simulink model "HalfBridgeRD"  (R2016a)
settings: Solver=VariableStepAuto  StartTime=0.0  StopTime=1.4e-6  RelTol=1e-3
values from neighbouring files (symbols this model uses):
  Dbot = 49    [HalfBridgeRDS.m]
  DelayBot = 50    [HalfBridgeRDS.m]
  DelayTop = 0    [HalfBridgeRDS.m]
  Dtop = 49    [HalfBridgeRDS.m]
  fsw = 1000e3    (= 1000000)    [HalfBridgeRDS.m]
  Rd = 25e-6    (= 2.5e-05)    [HalfBridgeRDS.m]
  Rg = 1    [HalfBridgeRDS.m]
  Rload = 10    [HalfBridgeRDS.m]
  Roff = 2    [HalfBridgeRDS.m]
  Ron = 12    [HalfBridgeRDS.m]
  Rs = 25e-6    (= 2.5e-05)    [HalfBridgeRDS.m]
libraries: elec_lib x28, fl_lib x14, nesl_utility x14
settings Model: Creator=ugurm  LastModifiedBy=ugurm

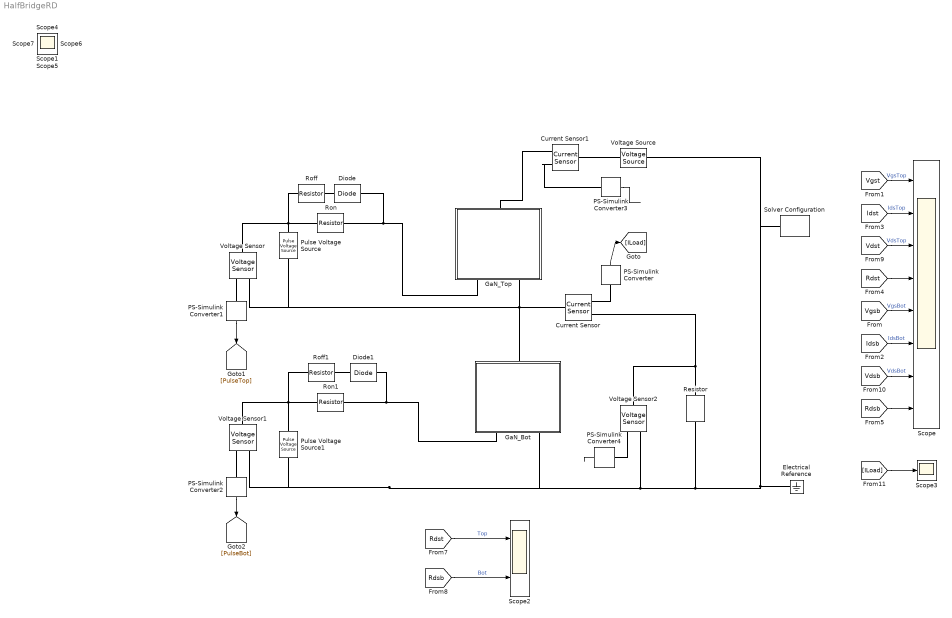
== system HalfBridgeRD ==
  Current Sensor : fl_lib/Electrical/Electrical Sensors/Current Sensor
  Current Sensor1 : fl_lib/Electrical/Electrical Sensors/Current Sensor
  Diode : elec_lib/Semiconductor Devices/Diode  ModelType=1  Vf=0.6 V  Ron=0.3 Ohm  Goff=1e-8 S  Rz=0.3 Ohm  Vz=50 V  C_PWL=5 pF  prmExp=1  I12=[ 0.0137 0.545 ] A  V12=[ 0.6 0.7 ] V  I1=0.0137 A  V1=0.6 V  RS=0.01 Ohm  IS=1e-12 A  Tmeas=25 degC  ec=1  BV=Inf V  C_param=1  CJ0=5 pF  VJ=1 V  Mgrad=0.5  Vvec=[ 0.1 10 100 ] V  Cvec=[ 3.5 1 0.4 ] pF  FC=0.5  Q_param=1  Irrm=-7.15 A  iF=4 A  didt=-750 A/us  trr=115 ns  TT=50 ns  tau=100 ns  T_param=1  IS_T2=1.25e-7 A  I1_T2=0.245 A  V1_T2=0.5 V  Tmeas2=125 degC  EG_param=1  EG=1.11 eV  XTI_param=1  XTI=3  dBVdT=0 V/K  Tdevice=25 degC  Rth=[ 0 10 ] K/W  thermal_mass_parameterization=1  thermal_mass=[ 0 1 ] J/K  thermal_time_constant=[ 0 10 ] s  thermal_mass_initial_temperatures=[ 25 25 ] degC
  Diode1 : elec_lib/Semiconductor Devices/Diode  ModelType=1  Vf=0.6 V  Ron=0.3 Ohm  Goff=1e-8 S  Rz=0.3 Ohm  Vz=50 V  C_PWL=5 pF  prmExp=1  I12=[ 0.0137 0.545 ] A  V12=[ 0.6 0.7 ] V  I1=0.0137 A  V1=0.6 V  RS=0.01 Ohm  IS=1e-12 A  Tmeas=25 degC  ec=1  BV=Inf V  C_param=1  CJ0=5 pF  VJ=1 V  Mgrad=0.5  Vvec=[ 0.1 10 100 ] V  Cvec=[ 3.5 1 0.4 ] pF  FC=0.5  Q_param=1  Irrm=-7.15 A  iF=4 A  didt=-750 A/us  trr=115 ns  TT=50 ns  tau=100 ns  T_param=1  IS_T2=1.25e-7 A  I1_T2=0.245 A  V1_T2=0.5 V  Tmeas2=125 degC  EG_param=1  EG=1.11 eV  XTI_param=1  XTI=3  dBVdT=0 V/K  Tdevice=25 degC  Rth=[ 0 10 ] K/W  thermal_mass_parameterization=1  thermal_mass=[ 0 1 ] J/K  thermal_time_constant=[ 0 10 ] s  thermal_mass_initial_temperatures=[ 25 25 ] degC
  Electrical Reference : fl_lib/Electrical/Electrical Elements/Electrical Reference
  GaN_Bot : Subsystem
  GaN_Top : Subsystem
  PS-Simulink Converter{,1..4} (5 alike) : nesl_utility/PS-Simulink Converter  PhysicalDomain=network_engine_domain  SubClassName=ps_output  LeftPortType=input  RightPortType=output  PseudoPeriodic=off  Frequencies=[]  Unit=1  AffineConversion=off
  Pulse Voltage Source : elec_lib/Additional Components/SPICE-Compatible Components/Sources/Pulse Voltage Source  V1=-3 V  V2=PulseAmplitude V  TD=DelayTop/(100*fsw) s  TR=1e-9 s  TF=1e-9 s  PW=Dtop/(100*fsw) s  PER=1/fsw s
  Pulse Voltage Source1 : elec_lib/Additional Components/SPICE-Compatible Components/Sources/Pulse Voltage Source  V1=-3 V  V2=PulseAmplitude V  TD=DelayBot/(100*fsw) s  TR=1e-9 s  TF=1e-9 s  PW=Dbot/(100*fsw) s  PER=1/fsw s
  Resistor : elec_lib/Passive Devices/Resistor  R=Rload Ohm  R_tol=5  enable_R_tol=0  tol_distribution=1  nSigma=4  enable_operating_limits=0  operating_limit_action=2  max_working_voltage=100 V  power_rating=1 W  enable_faults=0  fault_action=1  R_faulted=Inf Ohm  enable_temporal_fault=0  t_fault=1 s  enable_behavioral_fault=0  max_permissible_current=1 A  t_fail_on_current=1 s  noise_mode=0  sample_time=0.001 s  repeatability=1  auto_seed=3802589887  user_seed=0  Tdevice=25 degC  alpha=0.00393 1/K  Tmeas=25 degC  thermal_mass=100 J/K  initial_temperature=25 degC  power_derating_T1=70 degC  power_derating_T2=155 degC  operating_temperature_range_vec=[ -50 150 ] degC
  Roff : elec_lib/Passive Devices/Resistor  R=Roff Ohm  R_tol=5  enable_R_tol=0  tol_distribution=1  nSigma=4  enable_operating_limits=0  operating_limit_action=2  max_working_voltage=100 V  power_rating=1 W  enable_faults=0  fault_action=1  R_faulted=Inf Ohm  enable_temporal_fault=0  t_fault=1 s  enable_behavioral_fault=0  max_permissible_current=1 A  t_fail_on_current=1 s  noise_mode=0  sample_time=0.001 s  repeatability=1  auto_seed=935450722  user_seed=0  Tdevice=25 degC  alpha=0.00393 1/K  Tmeas=25 degC  thermal_mass=100 J/K  initial_temperature=25 degC  power_derating_T1=70 degC  power_derating_T2=155 degC  operating_temperature_range_vec=[ -50 150 ] degC
  Roff1 : elec_lib/Passive Devices/Resistor  R=Roff Ohm  R_tol=5  enable_R_tol=0  tol_distribution=1  nSigma=4  enable_operating_limits=0  operating_limit_action=2  max_working_voltage=100 V  power_rating=1 W  enable_faults=0  fault_action=1  R_faulted=Inf Ohm  enable_temporal_fault=0  t_fault=1 s  enable_behavioral_fault=0  max_permissible_current=1 A  t_fail_on_current=1 s  noise_mode=0  sample_time=0.001 s  repeatability=1  auto_seed=1550577895  user_seed=0  Tdevice=25 degC  alpha=0.00393 1/K  Tmeas=25 degC  thermal_mass=100 J/K  initial_temperature=25 degC  power_derating_T1=70 degC  power_derating_T2=155 degC  operating_temperature_range_vec=[ -50 150 ] degC
  Ron : elec_lib/Passive Devices/Resistor  R=Ron Ohm  R_tol=5  enable_R_tol=0  tol_distribution=1  nSigma=4  enable_operating_limits=0  operating_limit_action=2  max_working_voltage=100 V  power_rating=1 W  enable_faults=0  fault_action=1  R_faulted=Inf Ohm  enable_temporal_fault=0  t_fault=1 s  enable_behavioral_fault=0  max_permissible_current=1 A  t_fail_on_current=1 s  noise_mode=0  sample_time=0.001 s  repeatability=1  auto_seed=782289965  user_seed=0  Tdevice=25 degC  alpha=0.00393 1/K  Tmeas=25 degC  thermal_mass=100 J/K  initial_temperature=25 degC  power_derating_T1=70 degC  power_derating_T2=155 degC  operating_temperature_range_vec=[ -50 150 ] degC
  Ron1 : elec_lib/Passive Devices/Resistor  R=Ron Ohm  R_tol=5  enable_R_tol=0  tol_distribution=1  nSigma=4  enable_operating_limits=0  operating_limit_action=2  max_working_voltage=100 V  power_rating=1 W  enable_faults=0  fault_action=1  R_faulted=Inf Ohm  enable_temporal_fault=0  t_fault=1 s  enable_behavioral_fault=0  max_permissible_current=1 A  t_fail_on_current=1 s  noise_mode=0  sample_time=0.001 s  repeatability=1  auto_seed=2664075559  user_seed=0  Tdevice=25 degC  alpha=0.00393 1/K  Tmeas=25 degC  thermal_mass=100 J/K  initial_temperature=25 degC  power_derating_T1=70 degC  power_derating_T2=155 degC  operating_temperature_range_vec=[ -50 150 ] degC
  Scope : Scope  NumInputPorts=8
  Scope2 : Scope  NumInputPorts=2
  Scope{1,3..7} (6 alike) : Scope
  Solver Configuration : nesl_utility/Solver Configuration  PhysicalDomain=network_engine_domain  SubClassName=solver  LeftPortType=input  RightPortType=generic  Accelerate=off  Tones=[]  Harmonics=[]  SimulateNoise=off  Profile=off  UseLocalSampling=off  EnableSwitchedLinearOptims=on  FrequencyDomain=off  UseCCode=off  RelTol=0.001  AbsTol=1e-06  MinStep=1e-09  ToWorkspace=off  RevertToSquareIcSolve=off  NumHomotopyIterations=100  PhasorMode=off  PhasorModeNumHarmonics=1  OverrideAbsTol=off  DoDC=off  ResidualTolerance=1e-09  UseLocalSolver=on  LocalSolverChoice=NE_BACKWARD_EULER_ADVANCER  LocalSolverSampleTime=SampleTime  DoFixedCost=on  MaxNonlinIter=3  MaxModeIter=2  LinearAlgebra=Sparse  DelaysMemoryBudget=1024  AutomaticFiltering=on  FilteringTimeConstant=0.001
  Voltage Sensor : fl_lib/Electrical/Electrical Sensors/Voltage Sensor
  Voltage Sensor1 : fl_lib/Electrical/Electrical Sensors/Voltage Sensor
  Voltage Sensor2 : fl_lib/Electrical/Electrical Sensors/Voltage Sensor
  Voltage Source : elec_lib/Sources/Voltage Source  dc_voltage=Vdc V  ac_voltage=0 V  ac_shift=0 deg  ac_frequency=60 Hz  noise_mode=0  PSD=0 V^2/Hz  sample_time=0.001 s  repeatability=1  auto_seed=79941259  user_seed=0
  wires:
  PS-Simulink Converter/1 -> [ILoad]
  PS-Simulink Converter1/1 -> [PulseTop]
  PS-Simulink Converter2/1 -> [PulseBot]
  [Rdst] -> Scope2/1  "Top"
  [Rdsb] -> Scope2/2  "Bot"
  [Idst] -> Scope/2  "IdsTop"
  [Vgst] -> Scope/1  "VgsTop"
  [Vdst] -> Scope/3  "VdsTop"
  [ILoad] -> Scope3/1
  PS-Simulink Converter3/1 -> ?
  PS-Simulink Converter4/1 -> ?
  [Vgsb] -> Scope/5  "VgsBot"
  [Idsb] -> Scope/6  "IdsBot"
  [Vdsb] -> Scope/7  "VdsBot"
  [Rdst] -> Scope/4
  [Rdsb] -> Scope/8
  connections:
  Roff/RConn1 -- Ron/RConn1 -- Voltage Sensor/LConn1 -- Pulse Voltage Source/LConn1
  Diode/LConn1 -- Ron/LConn1 -- GaN_Top/LConn1
  Roff/LConn1 -- Diode/RConn1
  GaN_Top/LConn2 -- GaN_Bot/RConn1 -- Current Sensor/LConn1 -- Voltage Sensor/RConn2 -- Pulse Voltage Source/RConn1
  Pulse Voltage Source1/LConn1 -- Voltage Sensor1/LConn1 -- Ron1/RConn1 -- Roff1/RConn1
  Diode1/LConn1 -- GaN_Bot/LConn1 -- Ron1/LConn1
  Roff1/LConn1 -- Diode1/RConn1
  GaN_Bot/LConn2 -- Voltage Sensor1/RConn2 -- Pulse Voltage Source1/RConn1 -- Electrical Reference/LConn1 -- Voltage Source/RConn1 -- Solver Configuration/RConn1 -- Resistor/RConn1 -- Voltage Sensor2/RConn2
  PS-Simulink Converter/LConn1 -- Current Sensor/RConn1
  PS-Simulink Converter1/LConn1 -- Voltage Sensor/RConn1
  PS-Simulink Converter2/LConn1 -- Voltage Sensor1/RConn1
  Resistor/LConn1 -- Voltage Sensor2/LConn1 -- Current Sensor/RConn2
  Current Sensor1/RConn1 -- PS-Simulink Converter3/LConn1
  Voltage Sensor2/RConn1 -- PS-Simulink Converter4/LConn1
  Current Sensor1/RConn2 -- GaN_Top/RConn1
  Current Sensor1/LConn1 -- Voltage Source/LConn1

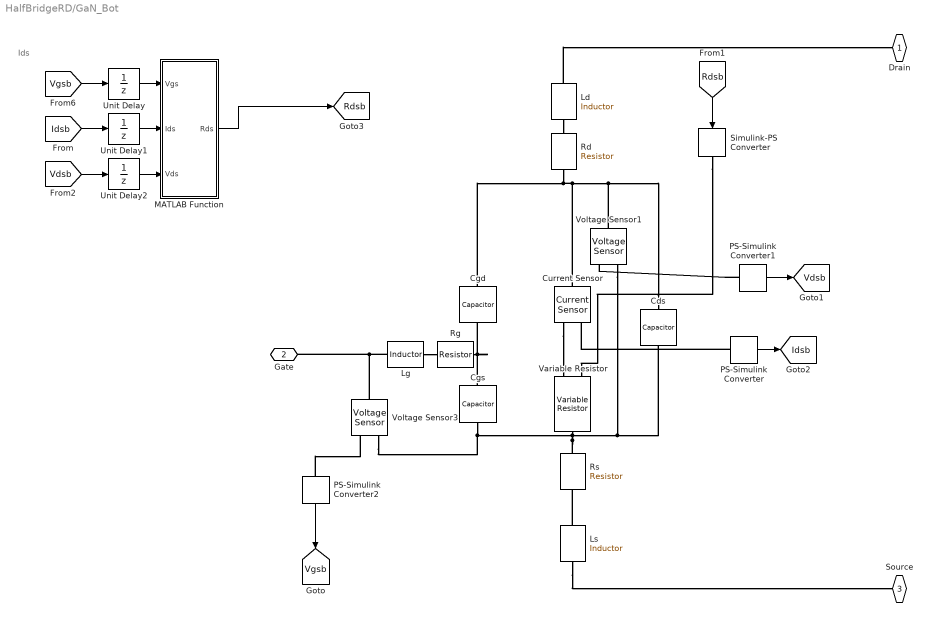
== system HalfBridgeRD/GaN_Bot ==
  note: Ids
  Cds : elec_lib/Passive Devices/Capacitor  enable_table=0  c=Cds F  Cvec=[ 1e-5 1e-6 ] F  Vvec=[ 0 10 ] V  CV_table_symmetry=1  C_tol=5  enable_C_tol=0  tol_distribution=1  nSigma=4  r=1e-6 Ohm  g=0 1/Ohm  initV=0 V  enable_operating_limits=0  operating_limit_action=2  max_working_voltage_range=[ -25 25 ] V  power_rating=1 W  enable_faults=0  fault_action=1  Cscale_faulted=100  R_faulted=0.001 Ohm  G_faulted=0 1/Ohm  tau_fault=0.001 s  enable_temporal_fault=0  t_fault=1 s  enable_behavioral_fault=0  max_permissible_voltage_range=[ -100 100 ] V  t_fail_on_voltage=1 s
  Cgd : elec_lib/Passive Devices/Capacitor  enable_table=0  c=Cgd F  Cvec=[ 1e-5 1e-6 ] F  Vvec=[ 0 10 ] V  CV_table_symmetry=1  C_tol=5  enable_C_tol=0  tol_distribution=1  nSigma=4  r=1e-6 Ohm  g=0 1/Ohm  initV=0 V  enable_operating_limits=0  operating_limit_action=2  max_working_voltage_range=[ -25 25 ] V  power_rating=1 W  enable_faults=0  fault_action=1  Cscale_faulted=100  R_faulted=0.001 Ohm  G_faulted=0 1/Ohm  tau_fault=0.001 s  enable_temporal_fault=0  t_fault=1 s  enable_behavioral_fault=0  max_permissible_voltage_range=[ -100 100 ] V  t_fail_on_voltage=1 s
  Cgs : elec_lib/Passive Devices/Capacitor  enable_table=0  c=Cgs F  Cvec=[ 1e-5 1e-6 ] F  Vvec=[ 0 10 ] V  CV_table_symmetry=1  C_tol=5  enable_C_tol=0  tol_distribution=1  nSigma=4  r=1e-6 Ohm  g=0 1/Ohm  initV=0 V  enable_operating_limits=0  operating_limit_action=2  max_working_voltage_range=[ -25 25 ] V  power_rating=1 W  enable_faults=0  fault_action=1  Cscale_faulted=100  R_faulted=0.001 Ohm  G_faulted=0 1/Ohm  tau_fault=0.001 s  enable_temporal_fault=0  t_fault=1 s  enable_behavioral_fault=0  max_permissible_voltage_range=[ -100 100 ] V  t_fail_on_voltage=1 s
  Current Sensor : fl_lib/Electrical/Electrical Sensors/Current Sensor
  Ld : elec_lib/Passive Devices/Inductor  l=Ld H  L_tol=5  enable_L_tol=0  tol_distribution=1  nSigma=4  r=0 Ohm  g=1e-9 1/Ohm  initI=0 A  enable_operating_limits=0  operating_limit_action=2  max_working_current=1 A  power_rating=1 W  enable_faults=0  fault_action=1  lambdaPercent=50  k_faulted=0.9999 Ohm  turnsShort=0  openCct=0  groundShort=0  groundShortG=0 1/Ohm  tau_fault=0.001 s  enable_temporal_fault=0  t_fault=1 s  enable_behavioral_fault=0  max_permissible_voltage=100 V  n_fail_on_voltage=1  max_permissible_current=1 A  t_fail_on_current=1 s
  Lg : elec_lib/Passive Devices/Inductor  l=Lg H  L_tol=5  enable_L_tol=0  tol_distribution=1  nSigma=4  r=0 Ohm  g=1e-9 1/Ohm  initI=0 A  enable_operating_limits=0  operating_limit_action=2  max_working_current=1 A  power_rating=1 W  enable_faults=0  fault_action=1  lambdaPercent=50  k_faulted=0.9999 Ohm  turnsShort=0  openCct=0  groundShort=0  groundShortG=0 1/Ohm  tau_fault=0.001 s  enable_temporal_fault=0  t_fault=1 s  enable_behavioral_fault=0  max_permissible_voltage=100 V  n_fail_on_voltage=1  max_permissible_current=1 A  t_fail_on_current=1 s
  Ls : elec_lib/Passive Devices/Inductor  l=Ls H  L_tol=5  enable_L_tol=0  tol_distribution=1  nSigma=4  r=0 Ohm  g=1e-9 1/Ohm  initI=0 A  enable_operating_limits=0  operating_limit_action=2  max_working_current=1 A  power_rating=1 W  enable_faults=0  fault_action=1  lambdaPercent=50  k_faulted=0.9999 Ohm  turnsShort=0  openCct=0  groundShort=0  groundShortG=0 1/Ohm  tau_fault=0.001 s  enable_temporal_fault=0  t_fault=1 s  enable_behavioral_fault=0  max_permissible_voltage=100 V  n_fail_on_voltage=1  max_permissible_current=1 A  t_fail_on_current=1 s
  MATLAB Function : MATLAB Function  TreatAsAtomicUnit=on
  PS-Simulink Converter : nesl_utility/PS-Simulink Converter  PhysicalDomain=network_engine_domain  SubClassName=ps_output  LeftPortType=input  RightPortType=output  PseudoPeriodic=off  Frequencies=[]  Unit=1  AffineConversion=off
  PS-Simulink Converter1 : nesl_utility/PS-Simulink Converter  PhysicalDomain=network_engine_domain  SubClassName=ps_output  LeftPortType=input  RightPortType=output  PseudoPeriodic=off  Frequencies=[]  Unit=1  AffineConversion=off
  PS-Simulink Converter2 : nesl_utility/PS-Simulink Converter  PhysicalDomain=network_engine_domain  SubClassName=ps_output  LeftPortType=input  RightPortType=output  PseudoPeriodic=off  Frequencies=[]  Unit=1  AffineConversion=off
  Rd : elec_lib/Passive Devices/Resistor  R=Rd Ohm  R_tol=5  enable_R_tol=0  tol_distribution=1  nSigma=4  enable_operating_limits=0  operating_limit_action=2  max_working_voltage=100 V  power_rating=1 W  enable_faults=0  fault_action=1  R_faulted=Inf Ohm  enable_temporal_fault=0  t_fault=1 s  enable_behavioral_fault=0  max_permissible_current=1 A  t_fail_on_current=1 s  noise_mode=0  sample_time=0.001 s  repeatability=1  auto_seed=2598415021  user_seed=0  Tdevice=25 degC  alpha=0.00393 1/K  Tmeas=25 degC  thermal_mass=100 J/K  initial_temperature=25 degC  power_derating_T1=70 degC  power_derating_T2=155 degC  operating_temperature_range_vec=[ -50 150 ] degC
  Rg : elec_lib/Passive Devices/Resistor  R=Rg Ohm  R_tol=5  enable_R_tol=0  tol_distribution=1  nSigma=4  enable_operating_limits=0  operating_limit_action=2  max_working_voltage=100 V  power_rating=1 W  enable_faults=0  fault_action=1  R_faulted=Inf Ohm  enable_temporal_fault=0  t_fault=1 s  enable_behavioral_fault=0  max_permissible_current=1 A  t_fail_on_current=1 s  noise_mode=0  sample_time=0.001 s  repeatability=1  auto_seed=1663206464  user_seed=0  Tdevice=25 degC  alpha=0.00393 1/K  Tmeas=25 degC  thermal_mass=100 J/K  initial_temperature=25 degC  power_derating_T1=70 degC  power_derating_T2=155 degC  operating_temperature_range_vec=[ -50 150 ] degC
  Rs : elec_lib/Passive Devices/Resistor  R=Rs Ohm  R_tol=5  enable_R_tol=0  tol_distribution=1  nSigma=4  enable_operating_limits=0  operating_limit_action=2  max_working_voltage=100 V  power_rating=1 W  enable_faults=0  fault_action=1  R_faulted=Inf Ohm  enable_temporal_fault=0  t_fault=1 s  enable_behavioral_fault=0  max_permissible_current=1 A  t_fail_on_current=1 s  noise_mode=0  sample_time=0.001 s  repeatability=1  auto_seed=610689199  user_seed=0  Tdevice=25 degC  alpha=0.00393 1/K  Tmeas=25 degC  thermal_mass=100 J/K  initial_temperature=25 degC  power_derating_T1=70 degC  power_derating_T2=155 degC  operating_temperature_range_vec=[ -50 150 ] degC
  Simulink-PS Converter : nesl_utility/Simulink-PS Converter  PhysicalDomain=network_engine_domain  SubClassName=ps_input  LeftPortType=input  RightPortType=output  PseudoPeriodic=off  Frequencies=[]  NoiseDistribution=none  NoiseParameters=[]  Unit=1  AffineConversion=off  InputFiltering=off  SimscapeFilterOrder=1  InputFilterTimeConstant=0.001  UdotUserProvided=1
  Unit Delay : UnitDelay  SampleTime=-1
  Unit Delay1 : UnitDelay  SampleTime=-1
  Unit Delay2 : UnitDelay  InitialCondition=1  SampleTime=-1
  Variable Resistor : fl_lib/Electrical/Electrical Elements/Variable Resistor  Rmin=0 Ohm  i_specify=off  i_priority=None  i=0 A  v_specify=off  v_priority=None  v=0 V
  Voltage Sensor1 : fl_lib/Electrical/Electrical Sensors/Voltage Sensor
  Voltage Sensor3 : fl_lib/Electrical/Electrical Sensors/Voltage Sensor
  Drain : PMIOPort  Port=1  Side=Right
  Gate : PMIOPort  Port=2  Side=Left
  Source : PMIOPort  Port=3  Side=Left
  tag scope: Idsb=global, Rdsb=global, Vdsb=global, Vgsb=global
  wires:
  [Rdsb] -> Simulink-PS Converter/1
  PS-Simulink Converter/1 -> [Idsb]
  PS-Simulink Converter2/1 -> [Vgsb]
  Unit Delay1/1 -> MATLAB Function/2(Ids)
  Unit Delay/1 -> MATLAB Function/1(Vgs)
  [Vgsb] -> Unit Delay/1
  [Idsb] -> Unit Delay1/1
  PS-Simulink Converter1/1 -> [Vdsb]
  Unit Delay2/1 -> MATLAB Function/3(Vds)
  [Vdsb] -> Unit Delay2/1
  MATLAB Function/1(Rds) -> [Rdsb]
  connections:
  Simulink-PS Converter/RConn1 -- Variable Resistor/LConn1
  PS-Simulink Converter/LConn1 -- Current Sensor/RConn1
  Current Sensor/RConn2 -- Variable Resistor/LConn2
  Ld/LConn1 -- Drain/RConn1
  Ls/RConn1 -- Source/RConn1
  PS-Simulink Converter2/LConn1 -- Voltage Sensor3/RConn1
  Voltage Sensor3/LConn1 -- Gate/RConn1 -- Lg/LConn1
  Ld/RConn1 -- Rd/LConn1
  Ls/LConn1 -- Rs/RConn1
  PS-Simulink Converter1/LConn1 -- Voltage Sensor1/RConn1
  Lg/RConn1 -- Rg/RConn1
  Cds/RConn1 -- Voltage Sensor1/RConn2 -- Cgs/RConn1 -- Voltage Sensor3/RConn2 -- Rs/LConn1 -- Variable Resistor/RConn1
  Rg/LConn1 -- Cgs/LConn1 -- Cgd/RConn1
  Cds/LConn1 -- Current Sensor/LConn1 -- Rd/RConn1 -- Cgd/LConn1 -- Voltage Sensor1/LConn1

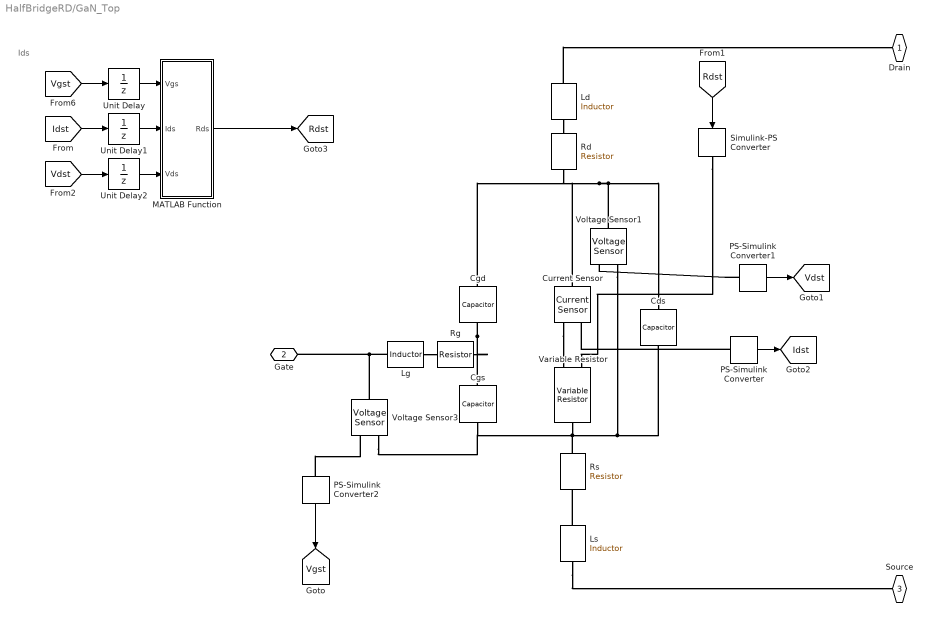
== system HalfBridgeRD/GaN_Top ==
  note: Ids
  Cds : elec_lib/Passive Devices/Capacitor  enable_table=0  c=Cds F  Cvec=[ 1e-5 1e-6 ] F  Vvec=[ 0 10 ] V  CV_table_symmetry=1  C_tol=5  enable_C_tol=0  tol_distribution=1  nSigma=4  r=1e-6 Ohm  g=0 1/Ohm  initV=0 V  enable_operating_limits=0  operating_limit_action=2  max_working_voltage_range=[ -25 25 ] V  power_rating=1 W  enable_faults=0  fault_action=1  Cscale_faulted=100  R_faulted=0.001 Ohm  G_faulted=0 1/Ohm  tau_fault=0.001 s  enable_temporal_fault=0  t_fault=1 s  enable_behavioral_fault=0  max_permissible_voltage_range=[ -100 100 ] V  t_fail_on_voltage=1 s
  Cgd : elec_lib/Passive Devices/Capacitor  enable_table=0  c=Cgd F  Cvec=[ 1e-5 1e-6 ] F  Vvec=[ 0 10 ] V  CV_table_symmetry=1  C_tol=5  enable_C_tol=0  tol_distribution=1  nSigma=4  r=1e-6 Ohm  g=0 1/Ohm  initV=0 V  enable_operating_limits=0  operating_limit_action=2  max_working_voltage_range=[ -25 25 ] V  power_rating=1 W  enable_faults=0  fault_action=1  Cscale_faulted=100  R_faulted=0.001 Ohm  G_faulted=0 1/Ohm  tau_fault=0.001 s  enable_temporal_fault=0  t_fault=1 s  enable_behavioral_fault=0  max_permissible_voltage_range=[ -100 100 ] V  t_fail_on_voltage=1 s
  Cgs : elec_lib/Passive Devices/Capacitor  enable_table=0  c=Cgs F  Cvec=[ 1e-5 1e-6 ] F  Vvec=[ 0 10 ] V  CV_table_symmetry=1  C_tol=5  enable_C_tol=0  tol_distribution=1  nSigma=4  r=1e-6 Ohm  g=0 1/Ohm  initV=0 V  enable_operating_limits=0  operating_limit_action=2  max_working_voltage_range=[ -25 25 ] V  power_rating=1 W  enable_faults=0  fault_action=1  Cscale_faulted=100  R_faulted=0.001 Ohm  G_faulted=0 1/Ohm  tau_fault=0.001 s  enable_temporal_fault=0  t_fault=1 s  enable_behavioral_fault=0  max_permissible_voltage_range=[ -100 100 ] V  t_fail_on_voltage=1 s
  Current Sensor : fl_lib/Electrical/Electrical Sensors/Current Sensor
  Ld : elec_lib/Passive Devices/Inductor  l=Ld H  L_tol=5  enable_L_tol=0  tol_distribution=1  nSigma=4  r=0 Ohm  g=1e-9 1/Ohm  initI=0 A  enable_operating_limits=0  operating_limit_action=2  max_working_current=1 A  power_rating=1 W  enable_faults=0  fault_action=1  lambdaPercent=50  k_faulted=0.9999 Ohm  turnsShort=0  openCct=0  groundShort=0  groundShortG=0 1/Ohm  tau_fault=0.001 s  enable_temporal_fault=0  t_fault=1 s  enable_behavioral_fault=0  max_permissible_voltage=100 V  n_fail_on_voltage=1  max_permissible_current=1 A  t_fail_on_current=1 s
  Lg : elec_lib/Passive Devices/Inductor  l=Lg H  L_tol=5  enable_L_tol=0  tol_distribution=1  nSigma=4  r=0 Ohm  g=1e-9 1/Ohm  initI=0 A  enable_operating_limits=0  operating_limit_action=2  max_working_current=1 A  power_rating=1 W  enable_faults=0  fault_action=1  lambdaPercent=50  k_faulted=0.9999 Ohm  turnsShort=0  openCct=0  groundShort=0  groundShortG=0 1/Ohm  tau_fault=0.001 s  enable_temporal_fault=0  t_fault=1 s  enable_behavioral_fault=0  max_permissible_voltage=100 V  n_fail_on_voltage=1  max_permissible_current=1 A  t_fail_on_current=1 s
  Ls : elec_lib/Passive Devices/Inductor  l=Ls H  L_tol=5  enable_L_tol=0  tol_distribution=1  nSigma=4  r=0 Ohm  g=1e-9 1/Ohm  initI=0 A  enable_operating_limits=0  operating_limit_action=2  max_working_current=1 A  power_rating=1 W  enable_faults=0  fault_action=1  lambdaPercent=50  k_faulted=0.9999 Ohm  turnsShort=0  openCct=0  groundShort=0  groundShortG=0 1/Ohm  tau_fault=0.001 s  enable_temporal_fault=0  t_fault=1 s  enable_behavioral_fault=0  max_permissible_voltage=100 V  n_fail_on_voltage=1  max_permissible_current=1 A  t_fail_on_current=1 s
  MATLAB Function : MATLAB Function  TreatAsAtomicUnit=on
  PS-Simulink Converter : nesl_utility/PS-Simulink Converter  PhysicalDomain=network_engine_domain  SubClassName=ps_output  LeftPortType=input  RightPortType=output  PseudoPeriodic=off  Frequencies=[]  Unit=1  AffineConversion=off
  PS-Simulink Converter1 : nesl_utility/PS-Simulink Converter  PhysicalDomain=network_engine_domain  SubClassName=ps_output  LeftPortType=input  RightPortType=output  PseudoPeriodic=off  Frequencies=[]  Unit=1  AffineConversion=off
  PS-Simulink Converter2 : nesl_utility/PS-Simulink Converter  PhysicalDomain=network_engine_domain  SubClassName=ps_output  LeftPortType=input  RightPortType=output  PseudoPeriodic=off  Frequencies=[]  Unit=1  AffineConversion=off
  Rd : elec_lib/Passive Devices/Resistor  R=Rd Ohm  R_tol=5  enable_R_tol=0  tol_distribution=1  nSigma=4  enable_operating_limits=0  operating_limit_action=2  max_working_voltage=100 V  power_rating=1 W  enable_faults=0  fault_action=1  R_faulted=Inf Ohm  enable_temporal_fault=0  t_fault=1 s  enable_behavioral_fault=0  max_permissible_current=1 A  t_fail_on_current=1 s  noise_mode=0  sample_time=0.001 s  repeatability=1  auto_seed=3861196639  user_seed=0  Tdevice=25 degC  alpha=0.00393 1/K  Tmeas=25 degC  thermal_mass=100 J/K  initial_temperature=25 degC  power_derating_T1=70 degC  power_derating_T2=155 degC  operating_temperature_range_vec=[ -50 150 ] degC
  Rg : elec_lib/Passive Devices/Resistor  R=Rg Ohm  R_tol=5  enable_R_tol=0  tol_distribution=1  nSigma=4  enable_operating_limits=0  operating_limit_action=2  max_working_voltage=100 V  power_rating=1 W  enable_faults=0  fault_action=1  R_faulted=Inf Ohm  enable_temporal_fault=0  t_fault=1 s  enable_behavioral_fault=0  max_permissible_current=1 A  t_fail_on_current=1 s  noise_mode=0  sample_time=0.001 s  repeatability=1  auto_seed=2688381633  user_seed=0  Tdevice=25 degC  alpha=0.00393 1/K  Tmeas=25 degC  thermal_mass=100 J/K  initial_temperature=25 degC  power_derating_T1=70 degC  power_derating_T2=155 degC  operating_temperature_range_vec=[ -50 150 ] degC
  Rs : elec_lib/Passive Devices/Resistor  R=Rs Ohm  R_tol=5  enable_R_tol=0  tol_distribution=1  nSigma=4  enable_operating_limits=0  operating_limit_action=2  max_working_voltage=100 V  power_rating=1 W  enable_faults=0  fault_action=1  R_faulted=Inf Ohm  enable_temporal_fault=0  t_fault=1 s  enable_behavioral_fault=0  max_permissible_current=1 A  t_fail_on_current=1 s  noise_mode=0  sample_time=0.001 s  repeatability=1  auto_seed=179614949  user_seed=0  Tdevice=25 degC  alpha=0.00393 1/K  Tmeas=25 degC  thermal_mass=100 J/K  initial_temperature=25 degC  power_derating_T1=70 degC  power_derating_T2=155 degC  operating_temperature_range_vec=[ -50 150 ] degC
  Simulink-PS Converter : nesl_utility/Simulink-PS Converter  PhysicalDomain=network_engine_domain  SubClassName=ps_input  LeftPortType=input  RightPortType=output  PseudoPeriodic=off  Frequencies=[]  NoiseDistribution=none  NoiseParameters=[]  Unit=1  AffineConversion=off  InputFiltering=off  SimscapeFilterOrder=1  InputFilterTimeConstant=0.001  UdotUserProvided=1
  Unit Delay : UnitDelay  SampleTime=-1
  Unit Delay1 : UnitDelay  SampleTime=-1
  Unit Delay2 : UnitDelay  InitialCondition=1  SampleTime=-1
  Variable Resistor : fl_lib/Electrical/Electrical Elements/Variable Resistor  Rmin=0 Ohm  i_specify=off  i_priority=None  i=0 A  v_specify=off  v_priority=None  v=0 V
  Voltage Sensor1 : fl_lib/Electrical/Electrical Sensors/Voltage Sensor
  Voltage Sensor3 : fl_lib/Electrical/Electrical Sensors/Voltage Sensor
  Drain : PMIOPort  Port=1  Side=Right
  Gate : PMIOPort  Port=2  Side=Left
  Source : PMIOPort  Port=3  Side=Left
  tag scope: Idst=global, Rdst=global, Vdst=global, Vgst=global
  wires:
  PS-Simulink Converter1/1 -> [Vdst]
  [Idst] -> Unit Delay1/1
  [Vgst] -> Unit Delay/1
  Unit Delay/1 -> MATLAB Function/1(Vgs)
  Unit Delay1/1 -> MATLAB Function/2(Ids)
  PS-Simulink Converter2/1 -> [Vgst]
  PS-Simulink Converter/1 -> [Idst]
  [Rdst] -> Simulink-PS Converter/1
  [Vdst] -> Unit Delay2/1
  Unit Delay2/1 -> MATLAB Function/3(Vds)
  MATLAB Function/1(Rds) -> [Rdst]
  connections:
  Cgd/LConn1 -- Rd/RConn1 -- Current Sensor/LConn1 -- Cds/LConn1 -- Voltage Sensor1/LConn1
  Cgd/RConn1 -- Cgs/LConn1 -- Rg/LConn1
  Rs/LConn1 -- Variable Resistor/RConn1 -- Voltage Sensor3/RConn2 -- Cgs/RConn1 -- Cds/RConn1 -- Voltage Sensor1/RConn2
  Lg/RConn1 -- Rg/RConn1
  PS-Simulink Converter1/LConn1 -- Voltage Sensor1/RConn1
  Ls/LConn1 -- Rs/RConn1
  Ld/RConn1 -- Rd/LConn1
  Lg/LConn1 -- Voltage Sensor3/LConn1 -- Gate/RConn1
  PS-Simulink Converter2/LConn1 -- Voltage Sensor3/RConn1
  Ls/RConn1 -- Source/RConn1
  Ld/LConn1 -- Drain/RConn1
  Current Sensor/RConn2 -- Variable Resistor/LConn2
  PS-Simulink Converter/LConn1 -- Current Sensor/RConn1
  Simulink-PS Converter/RConn1 -- Variable Resistor/LConn1

== matlab function HalfBridgeRD/GaN_Bot/MATLAB Function ==
  data: Vgs input; Rds output; Ids input; Vds input
function Rds = fcn(Vgs,Ids,Vds)
%#codegen
K1 = 0.283;
b1 = 2.035;
c1 = 0.124;
d1 = 1.159;
e1 = -0.204;
m1 = 30.972;
n1 = -4.48;
K2 = 7.114;
b2 = 2.054;
c2 = 0.153;
Vgd = Vgs - Vds;
if Ids>0
    Rds = 1/((K1*log(1+exp((Vgs-b1)/c1)))*(m1+n1*Vgs)-(d1+e1*Vgs)*Ids);
else
    Rds = 1/((K2*log(1+exp((Vgd-b2)/c2)))+Ids);
end
if Rds<0
    Rds = Rds*-1;
end

== matlab function HalfBridgeRD/GaN_Top/MATLAB Function ==
  data: Vgs input; Rds output; Ids input; Vds input
function Rds = fcn(Vgs,Ids,Vds)
%#codegen
K1 = 0.283;
b1 = 2.035;
c1 = 0.124;
d1 = 1.159;
e1 = -0.204;
m1 = 30.972;
n1 = -4.48;
K2 = 7.114;
b2 = 2.054;
c2 = 0.153;
Vgd = Vgs - Vds;

if Ids>0
    Rds = 1/((K1*log(1+exp((Vgs-b1)/c1)))*(m1+n1*Vgs)-(d1+e1*Vgs)*Ids);
else
    Rds = 1/((K2*log(1+exp((Vgd-b2)/c2)))+Ids);
end
